simulink model "ModeloEJ1"  (R2018b)
settings: Solver=VariableStepAuto  StartTime=0.0  StopTime=50  RelTol=1e-3
values from neighbouring files (symbols this model uses):
  A = Ag    [Example_VehicleSteering_Integral_action.m]
  B = Bg    [Example_VehicleSteering_Integral_action.m]
  C = eye(3)    [Example_VehicleSteering_Integral_action.m]
  K = [p - ap] * Wr_tilde * Wr^(-1)    [Example_VehicleSteering_Integral_action.m]
  kr = 1    [Example_VehicleSteering_Integral_action.m]
undefined symbols (not defined in the file or in its folder): d
settings Model: Creator=Acer  LastModifiedBy=Acer

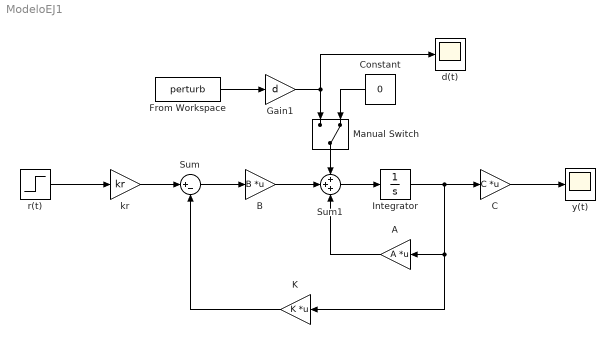
== system ModeloEJ1 ==
  A : Gain  Gain=A  Multiplication=Matrix(K*u) (u vector)
  B : Gain  Gain=B  Multiplication=Matrix(K*u) (u vector)
  C : Gain  Gain=C  Multiplication=Matrix(K*u) (u vector)
  Constant : Constant  Value=0
  From Workspace : FromWorkspace  VariableName=perturb  SampleTime=0  OutputAfterFinalValue=Setting to zero
  Gain1 : Gain  Gain=d
  Integrator : Integrator
  K : Gain  Gain=K  Multiplication=Matrix(K*u) (u vector)
  Manual Switch : ManualSwitch  CurrentSetting=0
  Sum : Sum  Inputs=|+-
  Sum1 : Sum  Inputs=+++
  d(t) : Scope
  kr : Gain  Gain=kr
  r(t) : Step  After=100  SampleTime=0
  y(t) : Scope
  wires:
  kr/1 -> Sum/1
  r(t)/1 -> kr/1
  Sum/1 -> B/1
  Sum1/1 -> Integrator/1
  Integrator/1 -> K/1, A/1, C/1
  C/1 -> y(t)/1
  K/1 -> Sum/2
  A/1 -> Sum1/3
  B/1 -> Sum1/2
  Manual Switch/1 -> Sum1/1
  Constant/1 -> Manual Switch/2
  Gain1/1 -> d(t)/1, Manual Switch/1
  From Workspace/1 -> Gain1/1
